simulink model "AllinOne2014a"  (R2014a)
settings: Solver=ode45  StartTime=0.0  StopTime=10.0  RelTol=1e-3
settings Model: DataDictionary=Struct.sldd  ParamWorkspaceSource=ReferencedWorkspace  Creator=89YY  LastModifiedBy=89YY
settings DebuggingCC: MergeDetectMultiDrivingBlocksExec=error

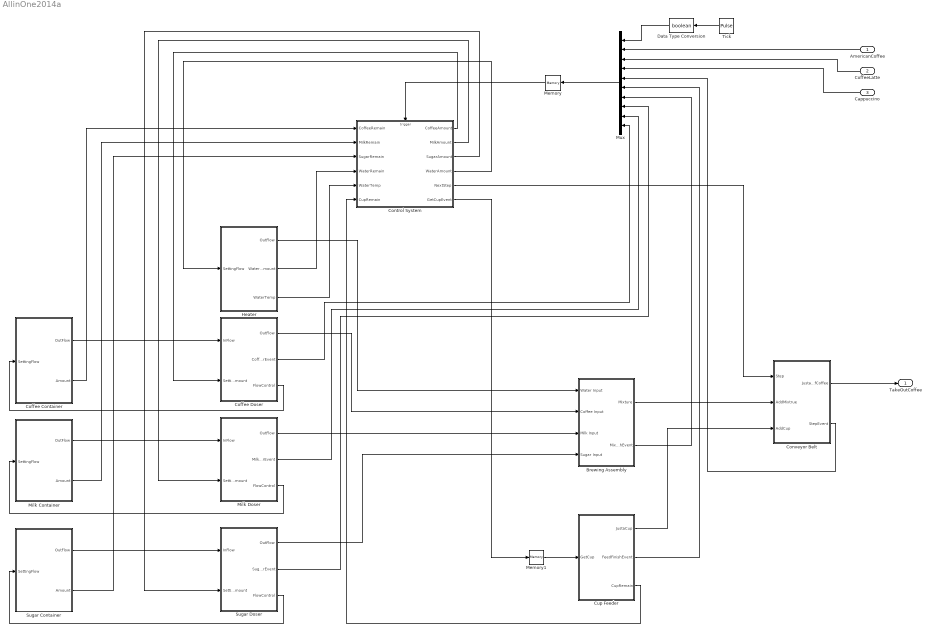
== system AllinOne2014a ==
  AmericanCoffee : Inport
  CoffeeLatte : Inport  Port=2
  Cappuccino : Inport  Port=3
  Brewing Assembly : Subsystem
  Coffee Container : Subsystem
  Coffee Doser : Subsystem
  Control System : Stateflow chart  TreatAsAtomicUnit=on
      settings: PermitHierarchicalResolution=ParametersOnly
  Conveyor Belt : Subsystem
  Cup Feeder : Subsystem
  Data Type Conversion : DataTypeConversion  OutDataTypeStr=boolean
  Heater : Subsystem
  Memory : Memory
  Memory1 : Memory
  Milk Container : Subsystem
  Milk Doser : Subsystem
  Mux : Mux  Inputs=10
  Sugar Container : Subsystem
  Sugar Doser : Subsystem
  Tick : DiscretePulseGenerator  PulseType=Time based  Period=0.01  PulseWidth=50
  TakeOutCoffee : Outport
  wires:
  Milk Container/1(OutFlow) -> Milk Doser/1(InFlow)
  Milk Doser/3(FlowControl) -> Milk Container/1(SettingFlow)
  Coffee Container/1(OutFlow) -> Coffee Doser/1(InFlow)
  Coffee Doser/3(FlowControl) -> Coffee Container/1(SettingFlow)
  Sugar Container/1(OutFlow) -> Sugar Doser/1(InFlow)
  Sugar Doser/3(FlowControl) -> Sugar Container/1(SettingFlow)
  Coffee Doser/1(OutFlow) -> Brewing Assembly/2(Coffee Input)
  Milk Doser/1(OutFlow) -> Brewing Assembly/3(Milk Input)
  Sugar Doser/1(OutFlow) -> Brewing Assembly/4(Sugar Input)
  Brewing Assembly/1(Mixture) -> Conveyor Belt/2(AddMixtrue)
  Cup Feeder/1(JustaCup) -> Conveyor Belt/3(AddCup)
  Coffee Container/2(Amount) -> Control System/1(CoffeeRemain)
  Milk Container/2(Amount) -> Control System/2(MilkRemain)
  Sugar Container/2(Amount) -> Control System/3(SugarRemain)
  Control System/6(GetCupEvent) -> Memory1/1
  Control System/1(CoffeeAmount) -> Coffee Doser/2(SettingAmount)
  Control System/2(MilkAmount) -> Milk Doser/2(SettingAmount)
  Control System/3(SugarAmount) -> Sugar Doser/2(SettingAmount)
  Coffee Doser/2(CoffeeDoserEvent) -> Mux/10
  Milk Doser/2(MilkDoserEvent) -> Mux/9
  Sugar Doser/2(SugarDoserEvent) -> Mux/8
  Control System/4(WaterAmount) -> Heater/1(SettingFlow)
  Cup Feeder/2(FeedFinishEvent) -> Mux/6
  Brewing Assembly/2(MixFinishEvent) -> Mux/7
  Conveyor Belt/2(StepEvent) -> Mux/5
  Control System/5(NextStep) -> Conveyor Belt/1(Step)
  Conveyor Belt/1(JustaCupofCoffee) -> TakeOutCoffee/1
  AmericanCoffee/1 -> Mux/2
  CoffeeLatte/1 -> Mux/3
  Cappuccino/1 -> Mux/4
  Mux/1 -> Memory/1
  Heater/1(OutFlow) -> Brewing Assembly/1(Water Input)
  Heater/2(WaterAmount) -> Control System/4(WaterRemain)
  Heater/3(WaterTemp) -> Control System/5(WaterTemp)
  Cup Feeder/3(CupRemain) -> Control System/6(CupRemain)
  Tick/1 -> Data Type Conversion/1
  Data Type Conversion/1 -> Mux/1
  Memory/1 -> Control System/Trigger
  Memory1/1 -> Cup Feeder/1(GetCup)

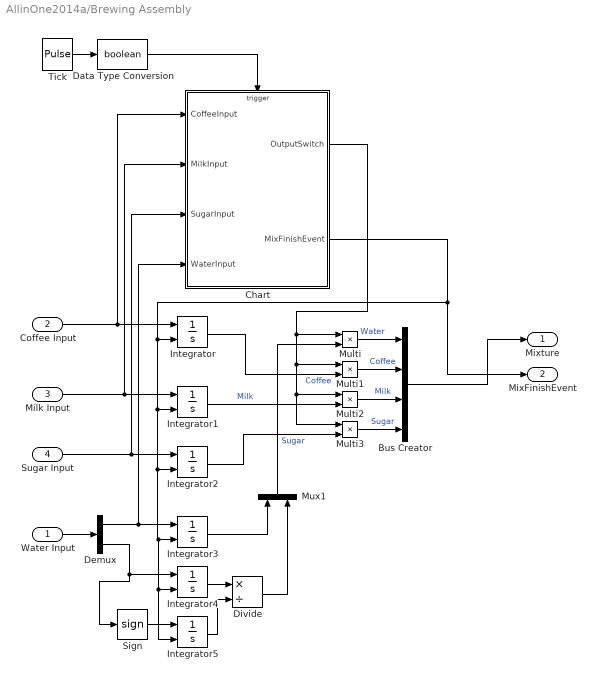
== system AllinOne2014a/Brewing Assembly ==
  Water Input : Inport
  Coffee Input : Inport  Port=2
  Milk Input : Inport  Port=3
  Sugar Input : Inport  Port=4
  Bus Creator : BusCreator  OutDataTypeStr=Bus: Mixtrue
  Chart : Stateflow chart  TreatAsAtomicUnit=on
      settings: PermitHierarchicalResolution=ParametersOnly
  Data Type Conversion : DataTypeConversion  OutDataTypeStr=boolean
  Demux : Demux  Outputs=2
  Divide : Product  Inputs=*/
  Integrator{,1..5} (6 alike) : Integrator  ExternalReset=rising
  Multi{,1..3} (4 alike) : Product  Inputs=**
  Mux1 : Mux  Inputs=2
  Sign : Signum
  Tick : DiscretePulseGenerator  PulseType=Time based  Period=0.01  PulseWidth=50
  Mixture : Outport  OutDataTypeStr=Bus: Mixtrue
  MixFinishEvent : Outport  Port=2
  wires:
  Tick/1 -> Data Type Conversion/1
  Data Type Conversion/1 -> Chart/Trigger
  Sugar Input/1 -> Integrator2/1, Chart/3(SugarInput)
  Demux/1 -> Chart/4(WaterInput), Integrator3/1
  Milk Input/1 -> Integrator1/1, Chart/2(MilkInput)
  Coffee Input/1 -> Integrator/1, Chart/1(CoffeeInput)
  Chart/2(MixFinishEvent) -> MixFinishEvent/1, Integrator5/2, Integrator4/2, Integrator3/2, Integrator2/2, Integrator1/2, Integrator/2
  Multi1/1 -> Bus Creator/2  "Coffee"
  Mux1/1 -> Multi/2
  Multi2/1 -> Bus Creator/3  "Milk"
  Multi3/1 -> Bus Creator/4  "Sugar"
  Bus Creator/1 -> Mixture/1
  Chart/1(OutputSwitch) -> Multi3/1, Multi2/1, Multi1/1, Multi/1
  Water Input/1 -> Demux/1
  Integrator3/1 -> Mux1/1
  Sign/1 -> Integrator5/1
  Demux/2 -> Sign/1, Integrator4/1
  Integrator4/1 -> Divide/1
  Integrator5/1 -> Divide/2
  Divide/1 -> Mux1/2
  Multi/1 -> Bus Creator/1  "Water"
  Integrator/1 -> Multi1/2  "Coffee"
  Integrator1/1 -> Multi2/2  "Milk"
  Integrator2/1 -> Multi3/2  "Sugar"

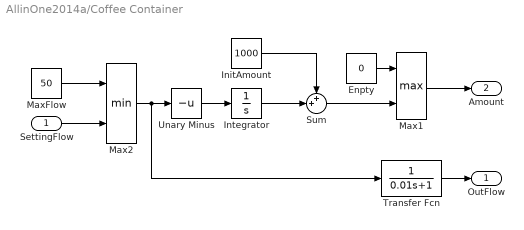
== system AllinOne2014a/Coffee Container ==
  SettingFlow : Inport
  Enpty : Constant  Value=0
  InitAmount : Constant  Value=1000
  Integrator : Integrator
  Max1 : MinMax  Function=max  Inputs=2
  Max2 : MinMax  Inputs=2  OutMin=[0]
  MaxFlow : Constant  Value=50
  Sum : Sum  Inputs=++|
  Transfer Fcn : TransferFcn  Denominator=[0.01 1]
  Unary Minus : UnaryMinus
  OutFlow : Outport
  Amount : Outport  Port=2
  wires:
  Unary Minus/1 -> Integrator/1
  Integrator/1 -> Sum/2
  SettingFlow/1 -> Max2/2
  InitAmount/1 -> Sum/1
  Max2/1 -> Transfer Fcn/1, Unary Minus/1
  MaxFlow/1 -> Max2/1
  Max1/1 -> Amount/1
  Sum/1 -> Max1/2
  Enpty/1 -> Max1/1
  Transfer Fcn/1 -> OutFlow/1

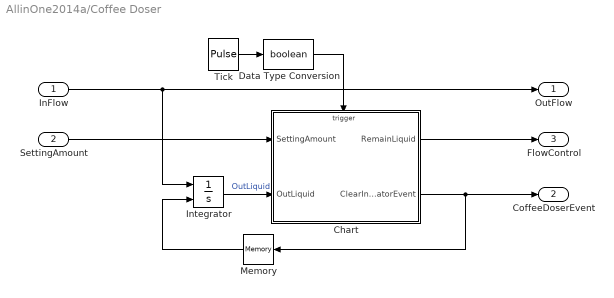
== system AllinOne2014a/Coffee Doser ==
  InFlow : Inport
  SettingAmount : Inport  Port=2
  Chart : Stateflow chart  RequirementInfo={} %GIDa_ffed56c2_cd34_4288_8248_c4489554cc95  TreatAsAtomicUnit=on
      settings: PermitHierarchicalResolution=ParametersOnly
  Data Type Conversion : DataTypeConversion  OutDataTypeStr=boolean
  Integrator : Integrator  ExternalReset=rising
  Memory : Memory
  Tick : DiscretePulseGenerator  PulseType=Time based  Period=0.01  PulseWidth=50
  OutFlow : Outport
  CoffeeDoserEvent : Outport  Port=2
  FlowControl : Outport  Port=3
  wires:
  SettingAmount/1 -> Chart/1(SettingAmount)
  Chart/1(RemainLiquid) -> FlowControl/1
  InFlow/1 -> OutFlow/1, Integrator/1
  Chart/2(ClearIntegratorEvent) -> Memory/1, CoffeeDoserEvent/1
  Integrator/1 -> Chart/2(OutLiquid)  "OutLiquid"
  Tick/1 -> Data Type Conversion/1
  Data Type Conversion/1 -> Chart/Trigger
  Memory/1 -> Integrator/2

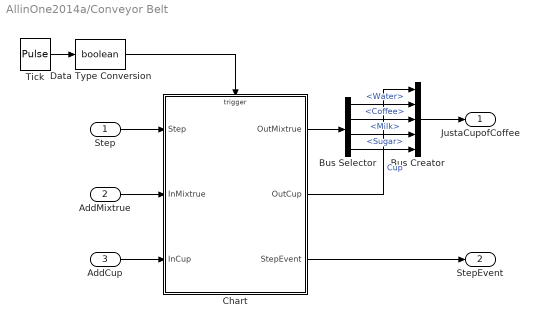
== system AllinOne2014a/Conveyor Belt ==
  Step : Inport
  AddMixtrue : Inport  Port=2
  AddCup : Inport  Port=3
  Bus Creator : BusCreator  Inputs=5
  Bus Selector : BusSelector  OutputSignals=Water,Coffee,Milk,Sugar
  Chart : Stateflow chart  TreatAsAtomicUnit=on
      settings: PermitHierarchicalResolution=ParametersOnly
  Data Type Conversion : DataTypeConversion  OutDataTypeStr=boolean
  Tick : DiscretePulseGenerator  PulseType=Time based  Period=0.01  PulseWidth=50
  JustaCupofCoffee : Outport  OutDataTypeStr=Bus: aCupofCoffee
  StepEvent : Outport  Port=2
  wires:
  Tick/1 -> Data Type Conversion/1
  Data Type Conversion/1 -> Chart/Trigger
  Chart/3(StepEvent) -> StepEvent/1
  AddCup/1 -> Chart/3(InCup)
  AddMixtrue/1 -> Chart/2(InMixtrue)
  Step/1 -> Chart/1(Step)
  Chart/1(OutMixtrue) -> Bus Selector/1
  Bus Selector/1 -> Bus Creator/2  "<Water>"
  Bus Selector/2 -> Bus Creator/3  "<Coffee>"
  Bus Selector/3 -> Bus Creator/4  "<Milk>"
  Bus Selector/4 -> Bus Creator/5  "<Sugar>"
  Chart/2(OutCup) -> Bus Creator/1  "Cup"
  Bus Creator/1 -> JustaCupofCoffee/1

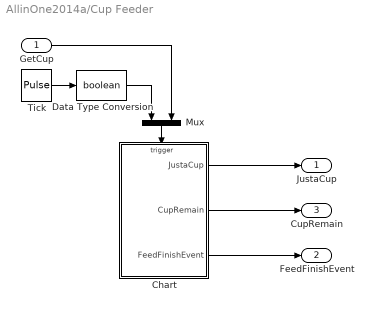
== system AllinOne2014a/Cup Feeder ==
  GetCup : Inport
  Chart : Stateflow chart  TreatAsAtomicUnit=on
      settings: PermitHierarchicalResolution=ParametersOnly
  Data Type Conversion : DataTypeConversion  OutDataTypeStr=boolean
  Mux : Mux  Inputs=2
  Tick : DiscretePulseGenerator  PulseType=Time based  Period=0.01  PulseWidth=50
  JustaCup : Outport
  FeedFinishEvent : Outport  Port=2
  CupRemain : Outport  Port=3
  wires:
  Chart/1(JustaCup) -> JustaCup/1
  Chart/2(CupRemain) -> CupRemain/1
  Chart/3(FeedFinishEvent) -> FeedFinishEvent/1
  GetCup/1 -> Mux/2
  Tick/1 -> Data Type Conversion/1
  Mux/1 -> Chart/Trigger
  Data Type Conversion/1 -> Mux/1

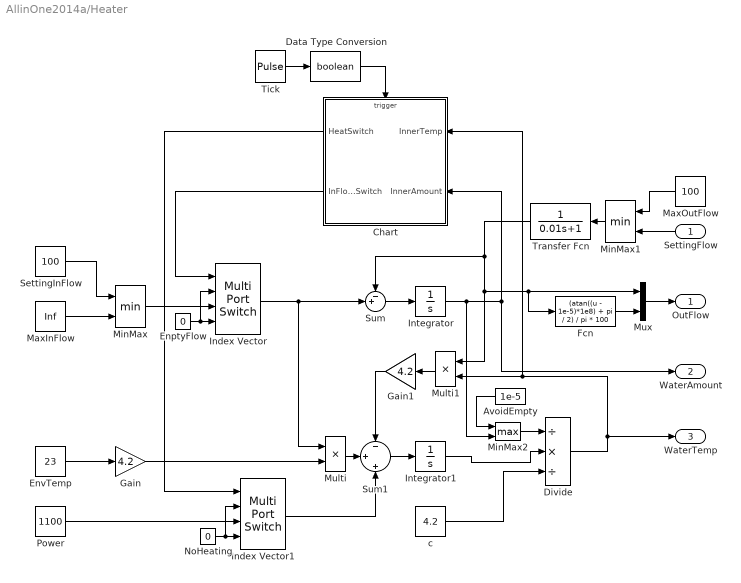
== system AllinOne2014a/Heater ==
  SettingFlow : Inport
  AvoidEmpty : Constant  Value=1e-5
  Chart : Stateflow chart  TreatAsAtomicUnit=on
      settings: PermitHierarchicalResolution=ParametersOnly
  Data Type Conversion : DataTypeConversion  OutDataTypeStr=boolean
  Divide : Product  Inputs=/*/
  EnptyFlow : Constant  Value=0
  EnvTemp : Constant  Value=23
  Fcn : Fcn  Expr=(atan((u - 1e-5)*1e8) + pi / 2) / pi * 100
  Gain : Gain  Gain=4.2
  Gain1 : Gain  Gain=4.2
  Index Vector : MultiPortSwitch  DataPortOrder=Zero-based contiguous  Inputs=2  DataPortForDefault=Additional data port  DiagnosticForDefault=None  zeroidx=on
  Index Vector1 : MultiPortSwitch  DataPortOrder=Zero-based contiguous  Inputs=2  DataPortForDefault=Additional data port  DiagnosticForDefault=None  zeroidx=on
  Integrator : Integrator
  Integrator1 : Integrator
  MaxInFlow : Constant  Value=Inf
  MaxOutFlow : Constant  Value=100
  MinMax : MinMax  Inputs=2
  MinMax1 : MinMax  Inputs=2
  MinMax2 : MinMax  Function=max  Inputs=2
  Multi : Product  Inputs=**
  Multi1 : Product  Inputs=**
  Mux : Mux  Inputs=2
  NoHeating : Constant  Value=0
  Power : Constant  Value=1100
  SettingInFlow : Constant  Value=100
  Sum : Sum  Inputs=-+|
  Sum1 : Sum  Inputs=-|+|+
  Tick : DiscretePulseGenerator  PulseType=Time based  Period=0.01  PulseWidth=50
  Transfer Fcn : TransferFcn  Denominator=[0.01 1]
  c : Constant  Value=4.2
  OutFlow : Outport
  WaterAmount : Outport  Port=2
  WaterTemp : Outport  Port=3
  wires:
  MaxInFlow/1 -> MinMax/2
  SettingInFlow/1 -> MinMax/1
  Sum/1 -> Integrator/1
  Sum1/1 -> Integrator1/1
  EnvTemp/1 -> Gain/1
  Integrator/1 -> MinMax2/2, WaterAmount/1, Chart/2(InnerAmount)
  Integrator1/1 -> Divide/2
  c/1 -> Divide/3
  Gain/1 -> Multi/2
  Multi/1 -> Sum1/2
  Index Vector/1 -> Multi/1, Sum/2
  EnptyFlow/1 -> Index Vector/2, Index Vector/4
  MinMax/1 -> Index Vector/3
  Chart/2(InFlowSwitch) -> Index Vector/1
  NoHeating/1 -> Index Vector1/2, Index Vector1/4
  Chart/1(HeatSwitch) -> Index Vector1/1
  Index Vector1/1 -> Sum1/3
  Power/1 -> Index Vector1/3
  MaxOutFlow/1 -> MinMax1/1
  SettingFlow/1 -> MinMax1/2
  MinMax1/1 -> Transfer Fcn/1
  Mux/1 -> OutFlow/1
  Transfer Fcn/1 -> Fcn/1, Mux/1, Multi1/1, Sum/1
  Tick/1 -> Data Type Conversion/1
  Data Type Conversion/1 -> Chart/Trigger
  Multi1/1 -> Gain1/1
  Gain1/1 -> Sum1/1
  MinMax2/1 -> Divide/1
  AvoidEmpty/1 -> MinMax2/1
  Divide/1 -> Multi1/2, Chart/1(InnerTemp), WaterTemp/1
  Fcn/1 -> Mux/2

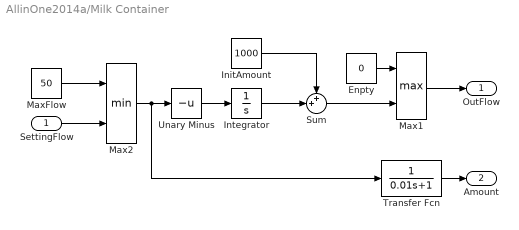
== system AllinOne2014a/Milk Container ==
  SettingFlow : Inport
  Enpty : Constant  Value=0
  InitAmount : Constant  Value=1000
  Integrator : Integrator
  Max1 : MinMax  Function=max  Inputs=2
  Max2 : MinMax  Inputs=2  OutMin=[0]
  MaxFlow : Constant  Value=50
  Sum : Sum  Inputs=++|
  Transfer Fcn : TransferFcn  Denominator=[0.01 1]
  Unary Minus : UnaryMinus
  OutFlow : Outport
  Amount : Outport  Port=2
  wires:
  Unary Minus/1 -> Integrator/1
  Integrator/1 -> Sum/2
  SettingFlow/1 -> Max2/2
  InitAmount/1 -> Sum/1
  Max2/1 -> Transfer Fcn/1, Unary Minus/1
  MaxFlow/1 -> Max2/1
  Max1/1 -> OutFlow/1
  Sum/1 -> Max1/2
  Enpty/1 -> Max1/1
  Transfer Fcn/1 -> Amount/1

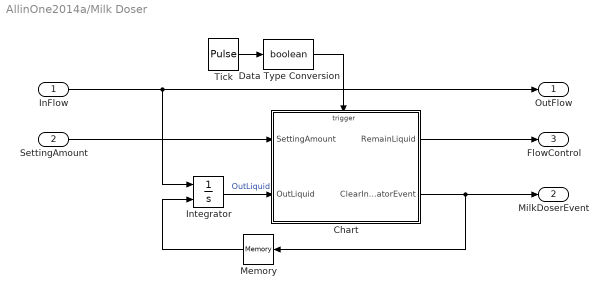
== system AllinOne2014a/Milk Doser ==
  InFlow : Inport
  SettingAmount : Inport  Port=2
  Chart : Stateflow chart  RequirementInfo={} %GIDa_551bb34e_10e7_4a73_950c_ffc9537d9666  TreatAsAtomicUnit=on
      settings: PermitHierarchicalResolution=ParametersOnly
  Data Type Conversion : DataTypeConversion  OutDataTypeStr=boolean
  Integrator : Integrator  ExternalReset=rising
  Memory : Memory
  Tick : DiscretePulseGenerator  PulseType=Time based  Period=0.01  PulseWidth=50
  OutFlow : Outport
  MilkDoserEvent : Outport  Port=2
  FlowControl : Outport  Port=3
  wires:
  SettingAmount/1 -> Chart/1(SettingAmount)
  Chart/1(RemainLiquid) -> FlowControl/1
  InFlow/1 -> OutFlow/1, Integrator/1
  Chart/2(ClearIntegratorEvent) -> Memory/1, MilkDoserEvent/1
  Integrator/1 -> Chart/2(OutLiquid)  "OutLiquid"
  Tick/1 -> Data Type Conversion/1
  Data Type Conversion/1 -> Chart/Trigger
  Memory/1 -> Integrator/2

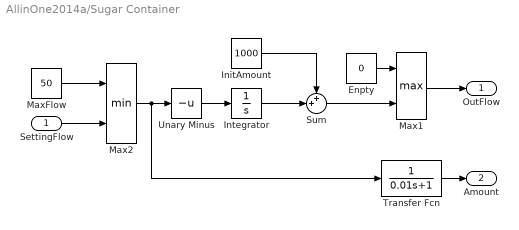
== system AllinOne2014a/Sugar Container ==
  SettingFlow : Inport
  Enpty : Constant  Value=0
  InitAmount : Constant  Value=1000
  Integrator : Integrator
  Max1 : MinMax  Function=max  Inputs=2
  Max2 : MinMax  Inputs=2  OutMin=[0]
  MaxFlow : Constant  Value=50
  Sum : Sum  Inputs=++|
  Transfer Fcn : TransferFcn  Denominator=[0.01 1]
  Unary Minus : UnaryMinus
  OutFlow : Outport
  Amount : Outport  Port=2
  wires:
  Unary Minus/1 -> Integrator/1
  Integrator/1 -> Sum/2
  SettingFlow/1 -> Max2/2
  InitAmount/1 -> Sum/1
  Max2/1 -> Transfer Fcn/1, Unary Minus/1
  MaxFlow/1 -> Max2/1
  Max1/1 -> OutFlow/1
  Sum/1 -> Max1/2
  Enpty/1 -> Max1/1
  Transfer Fcn/1 -> Amount/1

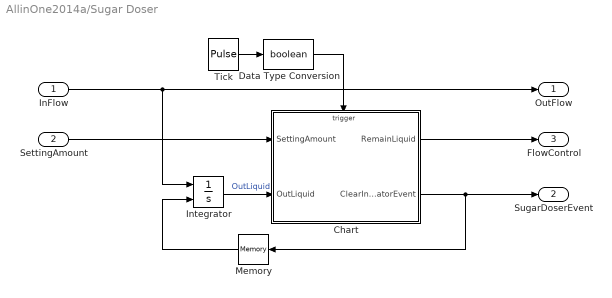
== system AllinOne2014a/Sugar Doser ==
  InFlow : Inport
  SettingAmount : Inport  Port=2
  Chart : Stateflow chart  RequirementInfo={} %GIDa_3f65ce12_bb97_4ef2_8d1d_79df95e5fb82  TreatAsAtomicUnit=on
      settings: PermitHierarchicalResolution=ParametersOnly
  Data Type Conversion : DataTypeConversion  OutDataTypeStr=boolean
  Integrator : Integrator  ExternalReset=rising
  Memory : Memory
  Tick : DiscretePulseGenerator  PulseType=Time based  Period=0.01  PulseWidth=50
  OutFlow : Outport
  SugarDoserEvent : Outport  Port=2
  FlowControl : Outport  Port=3
  wires:
  SettingAmount/1 -> Chart/1(SettingAmount)
  Chart/1(RemainLiquid) -> FlowControl/1
  InFlow/1 -> OutFlow/1, Integrator/1
  Chart/2(ClearIntegratorEvent) -> Memory/1, SugarDoserEvent/1
  Integrator/1 -> Chart/2(OutLiquid)  "OutLiquid"
  Tick/1 -> Data Type Conversion/1
  Data Type Conversion/1 -> Chart/Trigger
  Memory/1 -> Integrator/2

== stateflow chart AllinOne2014a/Conveyor Belt/Chart ==
  settings: executeAtInitialization=1  initializeOutput=1
  state MixtrueMonitor [parallel]
    settings: executionOrder=2
    state Waiting
    state Adding
      en:
      LocalMixtrue = InMixtrue
    MixtrueMonitor.Waiting -> MixtrueMonitor.Adding : [InMixtrue.Coffee > eps && ...
        | abs(CupLocation - 50) < 5]
    (default) -> MixtrueMonitor.Waiting
    MixtrueMonitor.Adding -> MixtrueMonitor.Waiting : [InMixtrue.Coffee > eps]
  state CupMonitor [parallel]
    settings: executionOrder=3
    state Waiting
    state Adding
      en:
      CupLocation = 0
    CupMonitor.Waiting -> CupMonitor.Adding : [InCup > eps && ...
        | CupLocation < 0]
    (default) -> CupMonitor.Waiting
    CupMonitor.Adding -> CupMonitor.Waiting : [InCup > eps]
  state CupTransmit [parallel]
    settings: executionOrder=1
    state Start
      en:CupLocation = -1
    state Running
    state Output
      en:
      OutMixtrue = LocalMixtrue;
      OutCup = 1;
      StepEvent;
      ex:
      StepEvent;
      OutMixtrue.Water = [0,0]';
      OutMixtrue.Coffee = 0;
      OutMixtrue.Milk = 0;
      OutMixtrue.Sugar = 0;
      OutCup = 0;
    state Prepare
    state Stepping
      en:
      CupLocation = CupLocation + Step
    Output -> Start : [after(10, Tick)]
    Start -> Running : [CupLocation >= 0]
    (default) -> Start
    Running -> Output [order 1] : [CupLocation >= 100]
    Stepping -> Running : [Step < eps]
    Running -> Prepare [order 2] : [Step > eps && CupLocation >= 0]
    Prepare -> Stepping : [after(Step, Tick)]
  data: Step input; CupLocation local; InMixtrue input Bus: Mixtrue; OutMixtrue output Bus: Mixtrue; InCup input; OutCup output; LocalMixtrue local Bus: Mixtrue
  events: Tick input RISING_EDGE_EVENT; StepEvent output EITHER_EDGE_EVENT

== stateflow chart AllinOne2014a/Milk Doser/Chart ==
  settings: sampleTime=TIMER  executeAtInitialization=1
  state Ready
  state Finish
  state Transmiting
    entry: TargetAmount = SettingAmount; RemainLiquid = TargetAmount / 3;
    exit: RemainLiquid = 0;
  (default) -> Ready
  Finish -> Ready : [after(5, Tick) && SettingAmount==0]
      | {
      | 	send(ClearIntegratorEvent);
      | }
  Ready -> Transmiting : [SettingAmount > 0]
  Transmiting -> Finish : [TargetAmount - OutLiquid <= 0]
      | {
      | 	send(ClearIntegratorEvent);
      | }
  data: SettingAmount input; RemainLiquid output; OutLiquid input; TargetAmount local
  events: ClearIntegratorEvent output EITHER_EDGE_EVENT; Tick input RISING_EDGE_EVENT

== stateflow chart AllinOne2014a/Sugar Doser/Chart ==
  settings: sampleTime=TIMER  executeAtInitialization=1
  state Ready
  state Finish
  state Transmiting
    entry: TargetAmount = SettingAmount; RemainLiquid = TargetAmount / 3;
    exit: RemainLiquid = 0;
  (default) -> Ready
  Finish -> Ready : [after(5, Tick) && SettingAmount==0]
      | {
      | 	send(ClearIntegratorEvent);
      | }
  Ready -> Transmiting : [SettingAmount > 0]
  Transmiting -> Finish : [TargetAmount - OutLiquid <= 0]
      | {
      | 	send(ClearIntegratorEvent);
      | }
  data: SettingAmount input; RemainLiquid output; OutLiquid input; TargetAmount local
  events: ClearIntegratorEvent output EITHER_EDGE_EVENT; Tick input RISING_EDGE_EVENT

== stateflow chart AllinOne2014a/Coffee Doser/Chart ==
  settings: sampleTime=TIMER  executeAtInitialization=1
  state Ready
  state Finish
  state Transmiting
    entry: TargetAmount = SettingAmount; RemainLiquid = TargetAmount / 3;
    exit: RemainLiquid = 0;
  (default) -> Ready
  Finish -> Ready : [after(5, Tick) && SettingAmount==0]
      | {
      | 	send(ClearIntegratorEvent);
      | }
  Ready -> Transmiting : [SettingAmount > 0]
  Transmiting -> Finish : [TargetAmount - OutLiquid <= 0]
      | {
      | 	send(ClearIntegratorEvent);
      | }
  data: SettingAmount input; RemainLiquid output; OutLiquid input; TargetAmount local
  events: ClearIntegratorEvent output EITHER_EDGE_EVENT; Tick input RISING_EDGE_EVENT

== stateflow chart AllinOne2014a/Cup Feeder/Chart ==
  settings: executeAtInitialization=1  initializeOutput=1
  state Ready
  state PutaCup
    entry:
    send(FeedFinishEvent);
    JustaCup = 1;
    CupAmount = CupAmount - 1;
    CupRemain = (CupAmount > 0);
    exit:
    JustaCup = 0;
    send(FeedFinishEvent);
  (default) -> Ready : {
      | 	CupAmount = 10;
      | 	CupRemain = (CupAmount > 0);
      | 	JustaCup = 0;
      | }
  PutaCup -> Ready : after(5, Tick)
  Ready -> PutaCup : NeedCupEvent[CupRemain > 0]
  data: JustaCup output; CupRemain output; CupAmount local
  events: FeedFinishEvent output EITHER_EDGE_EVENT; Tick input RISING_EDGE_EVENT; NeedCupEvent input RISING_EDGE_EVENT

== stateflow chart AllinOne2014a/Heater/Chart ==
  state InFlow [parallel]
    settings: executionOrder=2
    state GetInFlow
      en: InFlowSwitch = 1
    state OFF
      en: InFlowSwitch = 0
    GetInFlow -> InFlow.OFF : [InnerAmount>2000]
    (default) -> InFlow.OFF
    InFlow.OFF -> GetInFlow : [InnerAmount<1900]
  state Heater [parallel]
    settings: executionOrder=1
    state Heating
      en: HeatSwitch = 1
    state OFF
      en: HeatSwitch = 0
    Heating -> Heater.OFF : [InnerTemp>82]
    (default) -> Heater.OFF
    Heater.OFF -> Heating : [InnerTemp<78]
  data: InnerTemp input; InnerAmount input; HeatSwitch output; InFlowSwitch output
  events: Tick input RISING_EDGE_EVENT

== stateflow chart AllinOne2014a/Brewing Assembly/Chart ==
  settings: executeAtInitialization=1  initializeOutput=1
  state WaterState [parallel]
    settings: executionOrder=1
    state Waiting
    state Adding
    state Finished
    (default) -> WaterState.Waiting
    WaterState.Finished -> WaterState.Waiting : LocalFinishEvent
    WaterState.Waiting -> WaterState.Adding : [WaterInput > 0]
    WaterState.Adding -> WaterState.Finished : [WaterInput < 1e-5]
  state CoffeeState [parallel]
    settings: executionOrder=2
    state Waiting
    state Adding
    state Finished
    (default) -> CoffeeState.Waiting
    CoffeeState.Finished -> CoffeeState.Waiting : LocalFinishEvent
    CoffeeState.Waiting -> CoffeeState.Adding : [CoffeeInput > 0]
    CoffeeState.Adding -> CoffeeState.Finished : [CoffeeInput < 1e-5]
  state MilkState [parallel]
    settings: executionOrder=3
    state Waiting
    state Adding
    state Finished
    (default) -> MilkState.Waiting
    MilkState.Finished -> MilkState.Waiting : LocalFinishEvent
    MilkState.Waiting -> MilkState.Adding : [MilkInput > 0]
    MilkState.Adding -> MilkState.Finished : [MilkInput < 1e-5]
  state SugarState [parallel]
    settings: executionOrder=4
    state Waiting
    state Adding
    state Finished
    (default) -> SugarState.Waiting
    SugarState.Finished -> SugarState.Waiting : LocalFinishEvent
    SugarState.Waiting -> SugarState.Adding : [SugarInput > 0]
    SugarState.Adding -> SugarState.Finished : [SugarInput < 1e-5]
  state Mix [parallel]
    settings: executionOrder=5
    state Waiting
    state Mixing
    state Output
      en:
      OutputSwitch = 1;
      ex:
      OutputSwitch = 0;
    state Finished
      en:
      MixFinishEvent;
      LocalFinishEvent;
    Mix.Waiting -> Mixing : [in(WaterState.Finished) && ...
        | in(CoffeeState.Finished) && ...
        | in(MilkState.Finished) && ...
        | in(SugarState.Finished)]
    Output -> Mix.Finished : after(5, Tick)
    Mixing -> Output : after(5, Tick)
    (default) -> Mix.Waiting : {OutputSwitch = 0;}
    Mix.Finished -> Mix.Waiting : [after(10,Tick) && ...
        | in(WaterState.Waiting) && ...
        | in(CoffeeState.Waiting) && ...
        | in(MilkState.Waiting) && ...
        | in(SugarState.Waiting)]/
        | {
        | 	MixFinishEvent;
        | }
  data: CoffeeInput input; MilkInput input; SugarInput input; WaterInput input; OutputSwitch output
  events: Tick input RISING_EDGE_EVENT; MixFinishEvent output EITHER_EDGE_EVENT; LocalFinishEvent local FUNCTION_CALL_EVENT

== stateflow chart AllinOne2014a/Control System ==
  state Init
    en:
    CoffeeAmount = 0;
    MilkAmount = 0;
    SugarAmount = 0;
    WaterAmount = 0;
    NextStep = 0;
  (default) -> Init
  data: CoffeeRemain input; MilkRemain input; SugarRemain input; CoffeeAmount output; MilkAmount output; SugarAmount output; WaterAmount output; NextStep output; WaterRemain input; WaterTemp input; CupRemain input
  events: Tick input RISING_EDGE_EVENT; AmericanCoffee input RISING_EDGE_EVENT; CoffeeLatte input RISING_EDGE_EVENT; Cappuccino input RISING_EDGE_EVENT; StepEvent input RISING_EDGE_EVENT; FeedFinishEvent input RISING_EDGE_EVENT; MixFinishEvent input RISING_EDGE_EVENT; SugarDoserEvent input RISING_EDGE_EVENT; MilkDoserEvent input RISING_EDGE_EVENT; CoffeeDoserEvent input RISING_EDGE_EVENT; GetCupEvent output EITHER_EDGE_EVENT
